simulink model "HANcoder_E407_TTA_Template_DS_V1"  (R2023a)
settings: Solver=FixedStepDiscrete  StartTime=0.0  StopTime=1  FixedStep=0.01  RelTol=1e-3
PreLoadFcn:
  | librarySetup
  | eval([bdroot,'_startup']) %Calling [modelName]_startup.m
values from neighbouring files (symbols this model uses):
  basic_cycle_duration_bc0 = TM_Reset_Board   + COMP_duration    (= 372)    [HANcoder_E407_TTA_Template_DS_V1_startup.m]    (also in HANcoder_E407_TTA_Template_DS_V2_startup.m; HANcoder_E407_TTA_Template_DS_V52_startup.m; HANcoder_E407_TTA_Template_DS_V5_startup.m; HANcoder_E407_TTA_Template_DS_V6_startup.m = 532)
  basic_cycle_duration_bc1 = basic_cycle_duration_bc0    (= 372)    [HANcoder_E407_TTA_Template_DS_V1_startup.m]    (also in HANcoder_E407_TTA_Template_DS_V2_startup.m; HANcoder_E407_TTA_Template_DS_V52_startup.m; HANcoder_E407_TTA_Template_DS_V5_startup.m; HANcoder_E407_TTA_Template_DS_V6_startup.m = 532)
  basic_cycle_duration_bc2 = basic_cycle_duration_bc0    (= 372)    [HANcoder_E407_TTA_Template_DS_V1_startup.m]    (also in HANcoder_E407_TTA_Template_DS_V2_startup.m; HANcoder_E407_TTA_Template_DS_V52_startup.m; HANcoder_E407_TTA_Template_DS_V5_startup.m; HANcoder_E407_TTA_Template_DS_V6_startup.m = 532)
  comm_delay_estimation1 = round(comm_delay_measured1*hardware_granularity/frequency_IRQ)    [HANcoder_E407_TTA_Template_DS_V1_startup.m]    (also in HANcoder_E407_TTA_Template_DS_V2_startup.m; HANcoder_E407_TTA_Template_DS_V52_startup.m; HANcoder_E407_TTA_Template_DS_V5_startup.m; HANcoder_E407_TTA_Template_DS_V6_startup.m)
  comm_delay_estimation2 = round(comm_delay_measured2*hardware_granularity/frequency_IRQ)    [HANcoder_E407_TTA_Template_DS_V1_startup.m]    (also in HANcoder_E407_TTA_Template_DS_V2_startup.m; HANcoder_E407_TTA_Template_DS_V52_startup.m; HANcoder_E407_TTA_Template_DS_V5_startup.m; HANcoder_E407_TTA_Template_DS_V6_startup.m)
  COMM_Period = 80    [HANcoder_E407_TTA_Template_DS_V1_startup.m]    (also in HANcoder_E407_TTA_Template_DS_V2_startup.m; HANcoder_E407_TTA_Template_DS_V52_startup.m; HANcoder_E407_TTA_Template_DS_V5_startup.m; HANcoder_E407_TTA_Template_DS_V6_startup.m = 120)
  COMM_Phase1 = Simulink.Parameter    [HANcoder_E407_TTA_Template_DS_V1_startup.m]    (also in HANcoder_E407_TTA_Template_DS_V2_startup.m; HANcoder_E407_TTA_Template_DS_V52_startup.m; HANcoder_E407_TTA_Template_DS_V5_startup.m; HANcoder_E407_TTA_Template_DS_V6_startup.m)
  COMM_Phase2 = Simulink.Parameter    [HANcoder_E407_TTA_Template_DS_V1_startup.m]    (also in HANcoder_E407_TTA_Template_DS_V2_startup.m; HANcoder_E407_TTA_Template_DS_V52_startup.m; HANcoder_E407_TTA_Template_DS_V5_startup.m; HANcoder_E407_TTA_Template_DS_V6_startup.m)
  COMM_Phase_init1 = Simulink.Parameter    [HANcoder_E407_TTA_Template_DS_V1_startup.m]    (also in HANcoder_E407_TTA_Template_DS_V2_startup.m; HANcoder_E407_TTA_Template_DS_V52_startup.m; HANcoder_E407_TTA_Template_DS_V5_startup.m; HANcoder_E407_TTA_Template_DS_V6_startup.m)
  COMM_Phase_init2 = Simulink.Parameter    [HANcoder_E407_TTA_Template_DS_V1_startup.m]    (also in HANcoder_E407_TTA_Template_DS_V2_startup.m; HANcoder_E407_TTA_Template_DS_V52_startup.m; HANcoder_E407_TTA_Template_DS_V5_startup.m; HANcoder_E407_TTA_Template_DS_V6_startup.m)
  COMP_duration = 4    [HANcoder_E407_TTA_Template_DS_V1_startup.m]    (also in HANcoder_E407_TTA_Template_DS_V2_startup.m; HANcoder_E407_TTA_Template_DS_V52_startup.m; HANcoder_E407_TTA_Template_DS_V5_startup.m; HANcoder_E407_TTA_Template_DS_V6_startup.m)
  frequency_IRQ = 100    [HANcoder_E407_TTA_Template_DS_V1_startup.m]    (also in HANcoder_E407_TTA_Template_DS_V2_startup.m; HANcoder_E407_TTA_Template_DS_V52_startup.m; HANcoder_E407_TTA_Template_DS_V5_startup.m; HANcoder_E407_TTA_Template_DS_V6_startup.m)
  idle_time_init = basic_cycle_duration_bc0 + basic_cycle_duration_bc1    (= 744)    [HANcoder_E407_TTA_Template_DS_V1_startup.m]    (also in HANcoder_E407_TTA_Template_DS_V2_startup.m; HANcoder_E407_TTA_Template_DS_V52_startup.m = 1116; HANcoder_E407_TTA_Template_DS_V5_startup.m = 1116; HANcoder_E407_TTA_Template_DS_V6_startup.m = 1596)
  LA_Clock_Gr = 1    [HANcoder_E407_TTA_Template_DS_V1_startup.m]    (also in HANcoder_E407_TTA_Template_DS_V2_startup.m; HANcoder_E407_TTA_Template_DS_V52_startup.m; HANcoder_E407_TTA_Template_DS_V5_startup.m; HANcoder_E407_TTA_Template_DS_V6_startup.m)
  LA_COMM_dly = 1    [HANcoder_E407_TTA_Template_DS_V1_startup.m]    (also in HANcoder_E407_TTA_Template_DS_V2_startup.m; HANcoder_E407_TTA_Template_DS_V52_startup.m; HANcoder_E407_TTA_Template_DS_V5_startup.m; HANcoder_E407_TTA_Template_DS_V6_startup.m)
  LA_COMM_Err = 1    [HANcoder_E407_TTA_Template_DS_V1_startup.m]    (also in HANcoder_E407_TTA_Template_DS_V2_startup.m; HANcoder_E407_TTA_Template_DS_V52_startup.m; HANcoder_E407_TTA_Template_DS_V5_startup.m; HANcoder_E407_TTA_Template_DS_V6_startup.m)
  LA_E_Desync = 1    [HANcoder_E407_TTA_Template_DS_V1_startup.m]    (also in HANcoder_E407_TTA_Template_DS_V2_startup.m; HANcoder_E407_TTA_Template_DS_V52_startup.m; HANcoder_E407_TTA_Template_DS_V5_startup.m; HANcoder_E407_TTA_Template_DS_V6_startup.m)
  LA_MEX_Flag = 1    [HANcoder_E407_TTA_Template_DS_V1_startup.m]    (also in HANcoder_E407_TTA_Template_DS_V2_startup.m; HANcoder_E407_TTA_Template_DS_V52_startup.m; HANcoder_E407_TTA_Template_DS_V5_startup.m; HANcoder_E407_TTA_Template_DS_V6_startup.m)
  LA_Task_Act = 1    [HANcoder_E407_TTA_Template_DS_V1_startup.m]    (also in HANcoder_E407_TTA_Template_DS_V2_startup.m; HANcoder_E407_TTA_Template_DS_V52_startup.m; HANcoder_E407_TTA_Template_DS_V5_startup.m; HANcoder_E407_TTA_Template_DS_V6_startup.m)
  Master_Role = 1    [HANcoder_E407_TTA_Template_DS_V1_startup.m]    (also in HANcoder_E407_TTA_Template_DS_V2_startup.m; HANcoder_E407_TTA_Template_DS_V52_startup.m; HANcoder_E407_TTA_Template_DS_V5_startup.m; HANcoder_E407_TTA_Template_DS_V6_startup.m)
  matrix_rows = 3    [HANcoder_E407_TTA_Template_DS_V1_startup.m]    (also in HANcoder_E407_TTA_Template_DS_V2_startup.m; HANcoder_E407_TTA_Template_DS_V52_startup.m; HANcoder_E407_TTA_Template_DS_V5_startup.m; HANcoder_E407_TTA_Template_DS_V6_startup.m)
  max_desync = 15    [HANcoder_E407_TTA_Template_DS_V1_startup.m]    (also in HANcoder_E407_TTA_Template_DS_V2_startup.m; HANcoder_E407_TTA_Template_DS_V52_startup.m; HANcoder_E407_TTA_Template_DS_V5_startup.m; HANcoder_E407_TTA_Template_DS_V6_startup.m)
  max_num_msgs_CAN1 = 2^Tx_bit_number-1    (= 7)    [HANcoder_E407_TTA_Template_DS_V1_startup.m]    (also in HANcoder_E407_TTA_Template_DS_V2_startup.m; HANcoder_E407_TTA_Template_DS_V52_startup.m; HANcoder_E407_TTA_Template_DS_V5_startup.m; HANcoder_E407_TTA_Template_DS_V6_startup.m)
  max_num_msgs_CAN2 = max_num_msgs_CAN1    (= 7)    [HANcoder_E407_TTA_Template_DS_V1_startup.m]    (also in HANcoder_E407_TTA_Template_DS_V2_startup.m; HANcoder_E407_TTA_Template_DS_V52_startup.m; HANcoder_E407_TTA_Template_DS_V5_startup.m; HANcoder_E407_TTA_Template_DS_V6_startup.m)
  min_desync = (-1)*max_desync    (= -15)    [HANcoder_E407_TTA_Template_DS_V1_startup.m]    (also in HANcoder_E407_TTA_Template_DS_V2_startup.m; HANcoder_E407_TTA_Template_DS_V52_startup.m; HANcoder_E407_TTA_Template_DS_V5_startup.m; HANcoder_E407_TTA_Template_DS_V6_startup.m)
  PotValue1_ID = 22    [HANcoder_E407_TTA_Template_DS_V1_startup.m]    (also in HANcoder_E407_TTA_Template_DS_V2_startup.m; HANcoder_E407_TTA_Template_DS_V52_startup.m; HANcoder_E407_TTA_Template_DS_V5_startup.m; HANcoder_E407_TTA_Template_DS_V6_startup.m)
  PotValue2_ID = 23    [HANcoder_E407_TTA_Template_DS_V1_startup.m]    (also in HANcoder_E407_TTA_Template_DS_V2_startup.m; HANcoder_E407_TTA_Template_DS_V52_startup.m; HANcoder_E407_TTA_Template_DS_V5_startup.m; HANcoder_E407_TTA_Template_DS_V6_startup.m)
  PotValue3_ID = 24    [HANcoder_E407_TTA_Template_DS_V1_startup.m]    (also in HANcoder_E407_TTA_Template_DS_V2_startup.m; HANcoder_E407_TTA_Template_DS_V52_startup.m; HANcoder_E407_TTA_Template_DS_V5_startup.m; HANcoder_E407_TTA_Template_DS_V6_startup.m)
  script_run = Simulink.Parameter    [HANcoder_E407_TTA_Template_DS_V1_startup.m]    (also in HANcoder_E407_TTA_Template_DS_V2_startup.m; HANcoder_E407_TTA_Template_DS_V52_startup.m; HANcoder_E407_TTA_Template_DS_V5_startup.m; HANcoder_E407_TTA_Template_DS_V6_startup.m)
  Slave_Role = 2    [HANcoder_E407_TTA_Template_DS_V1_startup.m]    (also in HANcoder_E407_TTA_Template_DS_V2_startup.m; HANcoder_E407_TTA_Template_DS_V52_startup.m; HANcoder_E407_TTA_Template_DS_V5_startup.m; HANcoder_E407_TTA_Template_DS_V6_startup.m)
  Sync_ID = 1    [HANcoder_E407_TTA_Template_DS_V1_startup.m]    (also in HANcoder_E407_TTA_Template_DS_V2_startup.m; HANcoder_E407_TTA_Template_DS_V52_startup.m; HANcoder_E407_TTA_Template_DS_V5_startup.m; HANcoder_E407_TTA_Template_DS_V6_startup.m)
  TM_Check_PotValue1 = TM_COMM_PotValue1 + COMM_duration    (= 174)    [HANcoder_E407_TTA_Template_DS_V1_startup.m]    (also in HANcoder_E407_TTA_Template_DS_V2_startup.m; HANcoder_E407_TTA_Template_DS_V52_startup.m; HANcoder_E407_TTA_Template_DS_V5_startup.m; HANcoder_E407_TTA_Template_DS_V6_startup.m = 254)
  TM_Check_PotValue2 = TM_COMM_PotValue2 + COMM_duration    (= 258)    [HANcoder_E407_TTA_Template_DS_V1_startup.m]    (also in HANcoder_E407_TTA_Template_DS_V2_startup.m; HANcoder_E407_TTA_Template_DS_V52_startup.m; HANcoder_E407_TTA_Template_DS_V5_startup.m; HANcoder_E407_TTA_Template_DS_V6_startup.m = 378)
  TM_Check_PotValue3 = TM_COMM_PotValue3 + COMM_duration    (= 342)    [HANcoder_E407_TTA_Template_DS_V1_startup.m]    (also in HANcoder_E407_TTA_Template_DS_V2_startup.m; HANcoder_E407_TTA_Template_DS_V52_startup.m; HANcoder_E407_TTA_Template_DS_V5_startup.m; HANcoder_E407_TTA_Template_DS_V6_startup.m = 502)
  TM_Check_Sync = TM_COMM_Sync   + COMM_duration    (= 80)    [HANcoder_E407_TTA_Template_DS_V1_startup.m]    (also in HANcoder_E407_TTA_Template_DS_V2_startup.m; HANcoder_E407_TTA_Template_DS_V52_startup.m; HANcoder_E407_TTA_Template_DS_V5_startup.m; HANcoder_E407_TTA_Template_DS_V6_startup.m = 120)
  TM_Check_TOuts = TM_Count_Vote3 + COMP_duration    (= 356)    [HANcoder_E407_TTA_Template_DS_V1_startup.m]    (also in HANcoder_E407_TTA_Template_DS_V2_startup.m; HANcoder_E407_TTA_Template_DS_V52_startup.m; HANcoder_E407_TTA_Template_DS_V5_startup.m; HANcoder_E407_TTA_Template_DS_V6_startup.m = 516)
  TM_Check_Trailer1Articulation = TM_COMM_Trailer1Articulation + COMM_duration    (= 170)    [HANcoder_E407_TTA_Template_DS_V1_startup.m]    (also in HANcoder_E407_TTA_Template_DS_V2_startup.m; HANcoder_E407_TTA_Template_DS_V52_startup.m; HANcoder_E407_TTA_Template_DS_V5_startup.m; HANcoder_E407_TTA_Template_DS_V6_startup.m = 250)
  TM_Check_Trailer2Articulation = TM_COMM_Trailer2Articulation + COMM_duration    (= 254)    [HANcoder_E407_TTA_Template_DS_V1_startup.m]    (also in HANcoder_E407_TTA_Template_DS_V2_startup.m; HANcoder_E407_TTA_Template_DS_V52_startup.m; HANcoder_E407_TTA_Template_DS_V5_startup.m; HANcoder_E407_TTA_Template_DS_V6_startup.m = 374)
  TM_Check_Vote1 = TM_COMM_Vote1  + COMM_duration    (= 172)    [HANcoder_E407_TTA_Template_DS_V1_startup.m]    (also in HANcoder_E407_TTA_Template_DS_V2_startup.m; HANcoder_E407_TTA_Template_DS_V52_startup.m; HANcoder_E407_TTA_Template_DS_V5_startup.m; HANcoder_E407_TTA_Template_DS_V6_startup.m = 252)
  TM_Check_Vote2 = TM_COMM_Vote2  + COMM_duration    (= 260)    [HANcoder_E407_TTA_Template_DS_V1_startup.m]    (also in HANcoder_E407_TTA_Template_DS_V2_startup.m; HANcoder_E407_TTA_Template_DS_V52_startup.m; HANcoder_E407_TTA_Template_DS_V5_startup.m; HANcoder_E407_TTA_Template_DS_V6_startup.m = 380)
  TM_Check_Vote3 = TM_COMM_Vote3  + COMM_duration    (= 348)    [HANcoder_E407_TTA_Template_DS_V1_startup.m]    (also in HANcoder_E407_TTA_Template_DS_V2_startup.m; HANcoder_E407_TTA_Template_DS_V52_startup.m; HANcoder_E407_TTA_Template_DS_V5_startup.m; HANcoder_E407_TTA_Template_DS_V6_startup.m = 508)
  TM_COMM_PotValue1 = TM_ReadPot + COMP_duration    (= 94)    [HANcoder_E407_TTA_Template_DS_V1_startup.m]    (also in HANcoder_E407_TTA_Template_DS_V2_startup.m; HANcoder_E407_TTA_Template_DS_V52_startup.m; HANcoder_E407_TTA_Template_DS_V5_startup.m; HANcoder_E407_TTA_Template_DS_V6_startup.m = 134)
  TM_COMM_PotValue2 = TM_Check_PotValue1 + COMP_duration    (= 178)    [HANcoder_E407_TTA_Template_DS_V1_startup.m]    (also in HANcoder_E407_TTA_Template_DS_V2_startup.m; HANcoder_E407_TTA_Template_DS_V52_startup.m; HANcoder_E407_TTA_Template_DS_V5_startup.m; HANcoder_E407_TTA_Template_DS_V6_startup.m = 258)
  TM_COMM_PotValue3 = TM_Check_PotValue2 + COMP_duration    (= 262)    [HANcoder_E407_TTA_Template_DS_V1_startup.m]    (also in HANcoder_E407_TTA_Template_DS_V2_startup.m; HANcoder_E407_TTA_Template_DS_V52_startup.m; HANcoder_E407_TTA_Template_DS_V5_startup.m; HANcoder_E407_TTA_Template_DS_V6_startup.m = 382)
  TM_COMM_Sync = basic_cycle_start    (= 0)    [HANcoder_E407_TTA_Template_DS_V1_startup.m]    (also in HANcoder_E407_TTA_Template_DS_V2_startup.m; HANcoder_E407_TTA_Template_DS_V52_startup.m; HANcoder_E407_TTA_Template_DS_V5_startup.m; HANcoder_E407_TTA_Template_DS_V6_startup.m)
  TM_COMM_Trailer1Articulation = TM_Update_LT_2 + COMP_duration    (= 90)    [HANcoder_E407_TTA_Template_DS_V1_startup.m]    (also in HANcoder_E407_TTA_Template_DS_V2_startup.m; HANcoder_E407_TTA_Template_DS_V52_startup.m; HANcoder_E407_TTA_Template_DS_V5_startup.m; HANcoder_E407_TTA_Template_DS_V6_startup.m = 130)
  TM_COMM_Trailer2Articulation = TM_Check_Trailer1Articulation + COMP_duration    (= 174)    [HANcoder_E407_TTA_Template_DS_V1_startup.m]    (also in HANcoder_E407_TTA_Template_DS_V2_startup.m; HANcoder_E407_TTA_Template_DS_V52_startup.m; HANcoder_E407_TTA_Template_DS_V5_startup.m; HANcoder_E407_TTA_Template_DS_V6_startup.m = 254)
  TM_COMM_Vote1 = TM_Vote_Dec    + COMP_duration    (= 92)    [HANcoder_E407_TTA_Template_DS_V1_startup.m]    (also in HANcoder_E407_TTA_Template_DS_V2_startup.m; HANcoder_E407_TTA_Template_DS_V52_startup.m; HANcoder_E407_TTA_Template_DS_V5_startup.m; HANcoder_E407_TTA_Template_DS_V6_startup.m = 132)
  TM_COMM_Vote2 = TM_Count_Vote1 + COMP_duration    (= 180)    [HANcoder_E407_TTA_Template_DS_V1_startup.m]    (also in HANcoder_E407_TTA_Template_DS_V2_startup.m; HANcoder_E407_TTA_Template_DS_V52_startup.m; HANcoder_E407_TTA_Template_DS_V5_startup.m; HANcoder_E407_TTA_Template_DS_V6_startup.m = 260)
  TM_COMM_Vote3 = TM_Count_Vote2 + COMP_duration    (= 268)    [HANcoder_E407_TTA_Template_DS_V1_startup.m]    (also in HANcoder_E407_TTA_Template_DS_V2_startup.m; HANcoder_E407_TTA_Template_DS_V52_startup.m; HANcoder_E407_TTA_Template_DS_V5_startup.m; HANcoder_E407_TTA_Template_DS_V6_startup.m = 388)
  TM_Count_Vote1 = TM_Check_Vote1 + COMP_duration    (= 176)    [HANcoder_E407_TTA_Template_DS_V1_startup.m]    (also in HANcoder_E407_TTA_Template_DS_V2_startup.m; HANcoder_E407_TTA_Template_DS_V52_startup.m; HANcoder_E407_TTA_Template_DS_V5_startup.m; HANcoder_E407_TTA_Template_DS_V6_startup.m = 256)
  TM_Count_Vote2 = TM_Check_Vote2 + COMP_duration    (= 264)    [HANcoder_E407_TTA_Template_DS_V1_startup.m]    (also in HANcoder_E407_TTA_Template_DS_V2_startup.m; HANcoder_E407_TTA_Template_DS_V52_startup.m; HANcoder_E407_TTA_Template_DS_V5_startup.m; HANcoder_E407_TTA_Template_DS_V6_startup.m = 384)
  TM_Count_Vote3 = TM_Check_Vote3 + COMP_duration    (= 352)    [HANcoder_E407_TTA_Template_DS_V1_startup.m]    (also in HANcoder_E407_TTA_Template_DS_V2_startup.m; HANcoder_E407_TTA_Template_DS_V52_startup.m; HANcoder_E407_TTA_Template_DS_V5_startup.m; HANcoder_E407_TTA_Template_DS_V6_startup.m = 512)
  TM_Data_bc0 = TM_COMM_Sync    (= 0)    [HANcoder_E407_TTA_Template_DS_V1_startup.m]    (also in HANcoder_E407_TTA_Template_DS_V2_startup.m; HANcoder_E407_TTA_Template_DS_V52_startup.m; HANcoder_E407_TTA_Template_DS_V5_startup.m; HANcoder_E407_TTA_Template_DS_V6_startup.m)
  TM_Data_bc1 = TM_Data_bc0(1:4)    [HANcoder_E407_TTA_Template_DS_V1_startup.m]    (also in HANcoder_E407_TTA_Template_DS_V2_startup.m; HANcoder_E407_TTA_Template_DS_V52_startup.m; HANcoder_E407_TTA_Template_DS_V5_startup.m; HANcoder_E407_TTA_Template_DS_V6_startup.m)
  TM_Data_bc2 = TM_Data_bc0(1:4)    [HANcoder_E407_TTA_Template_DS_V1_startup.m]    (also in HANcoder_E407_TTA_Template_DS_V2_startup.m; HANcoder_E407_TTA_Template_DS_V52_startup.m; HANcoder_E407_TTA_Template_DS_V5_startup.m; HANcoder_E407_TTA_Template_DS_V6_startup.m)
  TM_New_Master = TM_Check_TOuts + COMP_duration    (= 360)    [HANcoder_E407_TTA_Template_DS_V1_startup.m]    (also in HANcoder_E407_TTA_Template_DS_V2_startup.m; HANcoder_E407_TTA_Template_DS_V52_startup.m; HANcoder_E407_TTA_Template_DS_V5_startup.m; HANcoder_E407_TTA_Template_DS_V6_startup.m = 520)
  TM_PotVote = TM_COMM_PotValue3 + COMP_duration    (= 266)    [HANcoder_E407_TTA_Template_DS_V1_startup.m]    (also in HANcoder_E407_TTA_Template_DS_V2_startup.m; HANcoder_E407_TTA_Template_DS_V52_startup.m; HANcoder_E407_TTA_Template_DS_V5_startup.m; HANcoder_E407_TTA_Template_DS_V6_startup.m = 386)
  TM_ReadPot = TM_Update_LT_2 + COMP_duration    (= 90)    [HANcoder_E407_TTA_Template_DS_V1_startup.m]    (also in HANcoder_E407_TTA_Template_DS_V2_startup.m; HANcoder_E407_TTA_Template_DS_V52_startup.m; HANcoder_E407_TTA_Template_DS_V5_startup.m; HANcoder_E407_TTA_Template_DS_V6_startup.m = 130)
  TM_Reset_Board = TM_Reset_Var   + COMP_duration    (= 368)    [HANcoder_E407_TTA_Template_DS_V1_startup.m]    (also in HANcoder_E407_TTA_Template_DS_V2_startup.m; HANcoder_E407_TTA_Template_DS_V52_startup.m; HANcoder_E407_TTA_Template_DS_V5_startup.m; HANcoder_E407_TTA_Template_DS_V6_startup.m = 528)
  TM_Reset_Var = TM_New_Master  + COMP_duration    (= 364)    [HANcoder_E407_TTA_Template_DS_V1_startup.m]    (also in HANcoder_E407_TTA_Template_DS_V2_startup.m; HANcoder_E407_TTA_Template_DS_V52_startup.m; HANcoder_E407_TTA_Template_DS_V5_startup.m; HANcoder_E407_TTA_Template_DS_V6_startup.m = 524)
  TM_Reset_Var_bc1 = TM_Data_bc1(end) + COMP_duration    [HANcoder_E407_TTA_Template_DS_V1_startup.m]    (also in HANcoder_E407_TTA_Template_DS_V2_startup.m; HANcoder_E407_TTA_Template_DS_V52_startup.m; HANcoder_E407_TTA_Template_DS_V5_startup.m; HANcoder_E407_TTA_Template_DS_V6_startup.m)
  TM_Reset_Var_bc1_2 = TM_Reset_Var_bc1 +2    [HANcoder_E407_TTA_Template_DS_V1_startup.m]    (also in HANcoder_E407_TTA_Template_DS_V2_startup.m; HANcoder_E407_TTA_Template_DS_V52_startup.m; HANcoder_E407_TTA_Template_DS_V5_startup.m; HANcoder_E407_TTA_Template_DS_V6_startup.m)
  TM_Type_bc0 = COMM    (= 0)    [HANcoder_E407_TTA_Template_DS_V1_startup.m]    (also in HANcoder_E407_TTA_Template_DS_V2_startup.m; HANcoder_E407_TTA_Template_DS_V52_startup.m; HANcoder_E407_TTA_Template_DS_V5_startup.m; HANcoder_E407_TTA_Template_DS_V6_startup.m)
  TM_Type_bc1 = TM_Type_bc0(1:4)    [HANcoder_E407_TTA_Template_DS_V1_startup.m]    (also in HANcoder_E407_TTA_Template_DS_V2_startup.m; HANcoder_E407_TTA_Template_DS_V52_startup.m; HANcoder_E407_TTA_Template_DS_V5_startup.m; HANcoder_E407_TTA_Template_DS_V6_startup.m)
  TM_Type_bc2 = TM_Type_bc0(1:4)    [HANcoder_E407_TTA_Template_DS_V1_startup.m]    (also in HANcoder_E407_TTA_Template_DS_V2_startup.m; HANcoder_E407_TTA_Template_DS_V52_startup.m; HANcoder_E407_TTA_Template_DS_V5_startup.m; HANcoder_E407_TTA_Template_DS_V6_startup.m)
  TM_Update_LT = TM_Check_Sync  + COMP_duration    (= 84)    [HANcoder_E407_TTA_Template_DS_V1_startup.m]    (also in HANcoder_E407_TTA_Template_DS_V2_startup.m; HANcoder_E407_TTA_Template_DS_V52_startup.m; HANcoder_E407_TTA_Template_DS_V5_startup.m; HANcoder_E407_TTA_Template_DS_V6_startup.m = 124)
  TM_Update_LT_2 = TM_Update_LT   + 2    (= 86)    [HANcoder_E407_TTA_Template_DS_V1_startup.m]    (also in HANcoder_E407_TTA_Template_DS_V2_startup.m; HANcoder_E407_TTA_Template_DS_V52_startup.m; HANcoder_E407_TTA_Template_DS_V5_startup.m; HANcoder_E407_TTA_Template_DS_V6_startup.m = 126)
  TM_Vote_Dec = TM_Update_LT   + COMP_duration    (= 88)    [HANcoder_E407_TTA_Template_DS_V1_startup.m]    (also in HANcoder_E407_TTA_Template_DS_V2_startup.m; HANcoder_E407_TTA_Template_DS_V52_startup.m; HANcoder_E407_TTA_Template_DS_V5_startup.m; HANcoder_E407_TTA_Template_DS_V6_startup.m = 128)
  Tractor_Board1 = 11    [HANcoder_E407_TTA_Template_DS_V1_startup.m]    (also in HANcoder_E407_TTA_Template_DS_V2_startup.m = 1; HANcoder_E407_TTA_Template_DS_V52_startup.m = 1; HANcoder_E407_TTA_Template_DS_V5_startup.m = 1; HANcoder_E407_TTA_Template_DS_V6_startup.m = 1)
  Trailer1_Articulation_ID = 31    [HANcoder_E407_TTA_Template_DS_V1_startup.m]    (also in HANcoder_E407_TTA_Template_DS_V2_startup.m; HANcoder_E407_TTA_Template_DS_V52_startup.m; HANcoder_E407_TTA_Template_DS_V5_startup.m; HANcoder_E407_TTA_Template_DS_V6_startup.m)
  Trailer1_Board1 = 2    [HANcoder_E407_TTA_Template_DS_V1_startup.m]    (also in HANcoder_E407_TTA_Template_DS_V2_startup.m = 4; HANcoder_E407_TTA_Template_DS_V52_startup.m = 4; HANcoder_E407_TTA_Template_DS_V5_startup.m = 4; HANcoder_E407_TTA_Template_DS_V6_startup.m = 4)
  Trailer1_Board2 = 3    [HANcoder_E407_TTA_Template_DS_V1_startup.m]    (also in HANcoder_E407_TTA_Template_DS_V2_startup.m = 5; HANcoder_E407_TTA_Template_DS_V52_startup.m = 5; HANcoder_E407_TTA_Template_DS_V5_startup.m = 5; HANcoder_E407_TTA_Template_DS_V6_startup.m = 5)
  Trailer1_Board3 = 4    [HANcoder_E407_TTA_Template_DS_V1_startup.m]    (also in HANcoder_E407_TTA_Template_DS_V2_startup.m = 6; HANcoder_E407_TTA_Template_DS_V52_startup.m = 6; HANcoder_E407_TTA_Template_DS_V5_startup.m = 6; HANcoder_E407_TTA_Template_DS_V6_startup.m = 6)
  Trailer2_Articulation_ID = 32    [HANcoder_E407_TTA_Template_DS_V1_startup.m]    (also in HANcoder_E407_TTA_Template_DS_V2_startup.m; HANcoder_E407_TTA_Template_DS_V52_startup.m; HANcoder_E407_TTA_Template_DS_V5_startup.m; HANcoder_E407_TTA_Template_DS_V6_startup.m)
  Trailer2_Board1 = 5    [HANcoder_E407_TTA_Template_DS_V1_startup.m]    (also in HANcoder_E407_TTA_Template_DS_V2_startup.m = 7; HANcoder_E407_TTA_Template_DS_V52_startup.m = 7; HANcoder_E407_TTA_Template_DS_V5_startup.m = 7; HANcoder_E407_TTA_Template_DS_V6_startup.m = 7)
  Trailer2_Board2 = 6    [HANcoder_E407_TTA_Template_DS_V1_startup.m]    (also in HANcoder_E407_TTA_Template_DS_V2_startup.m = 8; HANcoder_E407_TTA_Template_DS_V52_startup.m = 8; HANcoder_E407_TTA_Template_DS_V5_startup.m = 8; HANcoder_E407_TTA_Template_DS_V6_startup.m = 8)
  Trailer2_Board3 = 7    [HANcoder_E407_TTA_Template_DS_V1_startup.m]    (also in HANcoder_E407_TTA_Template_DS_V2_startup.m = 9; HANcoder_E407_TTA_Template_DS_V52_startup.m = 9; HANcoder_E407_TTA_Template_DS_V5_startup.m = 9; HANcoder_E407_TTA_Template_DS_V6_startup.m = 9)
  Vote1_ID = 11    [HANcoder_E407_TTA_Template_DS_V1_startup.m]    (also in HANcoder_E407_TTA_Template_DS_V2_startup.m; HANcoder_E407_TTA_Template_DS_V52_startup.m; HANcoder_E407_TTA_Template_DS_V5_startup.m; HANcoder_E407_TTA_Template_DS_V6_startup.m)
  Vote2_ID = 12    [HANcoder_E407_TTA_Template_DS_V1_startup.m]    (also in HANcoder_E407_TTA_Template_DS_V2_startup.m; HANcoder_E407_TTA_Template_DS_V52_startup.m; HANcoder_E407_TTA_Template_DS_V5_startup.m; HANcoder_E407_TTA_Template_DS_V6_startup.m)
  Vote3_ID = 13    [HANcoder_E407_TTA_Template_DS_V1_startup.m]    (also in HANcoder_E407_TTA_Template_DS_V2_startup.m; HANcoder_E407_TTA_Template_DS_V52_startup.m; HANcoder_E407_TTA_Template_DS_V5_startup.m; HANcoder_E407_TTA_Template_DS_V6_startup.m)
undefined symbols (not defined in the file or in its folder): A0, A1, A2, A3, A4, A5, CON2, CON4, D10, D12, D13, D8, D9
libraries: hdlsllib x164, HANcoder_STM32_Target x28, simulink x12, simulink_extras x1, dspstat3 x1
(part 5 of 34)

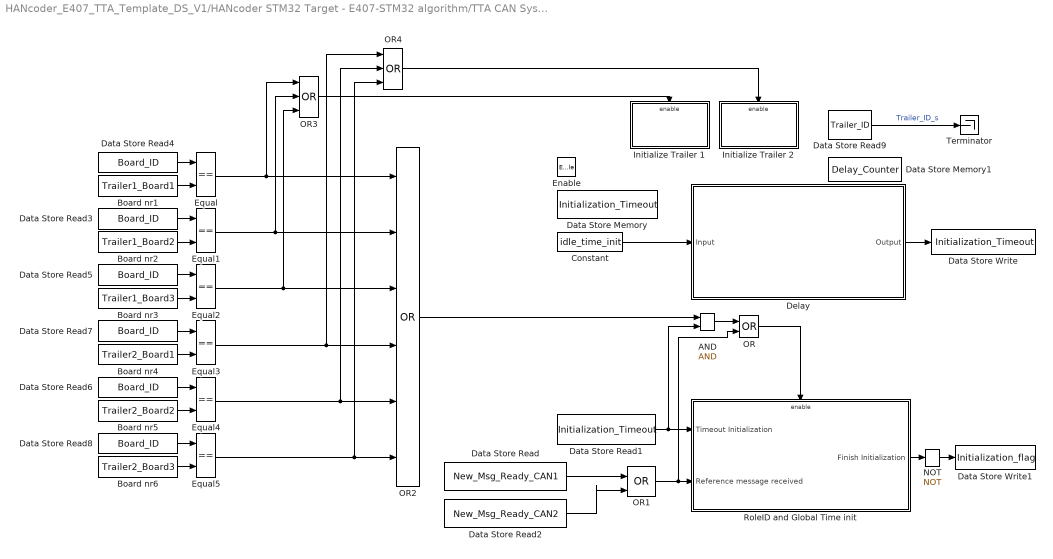
== system HANcoder_E407_TTA_Template_DS_V1/HANcoder STM32 Target - E407-STM32 algorithm/TTA CAN System/TTA System/Initialization ==
  Enable : EnablePort  PropagateVarSize=During execution
  AND : Logic  IconShape=distinctive  AllPortsSameDT=off  OutDataTypeStr=boolean
  Board nr1 : Constant  Value=Trailer1_Board1
  Board nr2 : Constant  Value=Trailer1_Board2
  Board nr3 : Constant  Value=Trailer1_Board3
  Board nr4 : Constant  Value=Trailer2_Board1
  Board nr5 : Constant  Value=Trailer2_Board2
  Board nr6 : Constant  Value=Trailer2_Board3
  Constant : Constant  Value=idle_time_init
  Data Store Memory : DataStoreMemory  DataStoreName=Initialization_Timeout  ReadBeforeWriteMsg=warning  WriteAfterWriteMsg=warning  WriteAfterReadMsg=warning  ShowAdditionalParam=off  OutDataTypeStr=boolean
  Data Store Memory1 : DataStoreMemory  DataStoreName=Delay_Counter  ReadBeforeWriteMsg=warning  WriteAfterWriteMsg=warning  WriteAfterReadMsg=warning  ShowAdditionalParam=off  OutDataTypeStr=double
  Data Store Read : DataStoreRead  DataStoreName=New_Msg_Ready_CAN1  IndexOptions=Index vector (dialog)  Indices=1  OutputSizes=1
  Data Store Read1 : DataStoreRead  DataStoreName=Initialization_Timeout  IndexOptions=Index vector (dialog)  Indices=1  OutputSizes=1
  Data Store Read2 : DataStoreRead  DataStoreName=New_Msg_Ready_CAN2  IndexOptions=Index vector (dialog)  Indices=1  OutputSizes=1
  Data Store Read{3..8} (6 alike) : DataStoreRead  DataStoreName=Board_ID  IndexOptions=Index vector (dialog)  Indices=1  OutputSizes=1
  Data Store Read9 : DataStoreRead  DataStoreName=Trailer_ID  IndexOptions=Index vector (dialog)  Indices=1  OutputSizes=1
  Data Store Write : DataStoreWrite  DataStoreName=Initialization_Timeout  IndexOptions=Index vector (dialog)  Indices=1  OutputSizes=1
  Data Store Write1 : DataStoreWrite  DataStoreName=Initialization_flag  IndexOptions=Index vector (dialog)  Indices=1  OutputSizes=1
  Delay : Subsystem
  Equal{,1..5} (6 alike) : RelationalOperator  Operator===  OutDataTypeStr=boolean  RndMeth=Simplest  InputSameDT=off
  Initialize Trailer 1 : Subsystem  TreatAsAtomicUnit=on
  Initialize Trailer 2 : Subsystem  TreatAsAtomicUnit=on
  NOT : Logic  Operator=NOT  IconShape=distinctive  AllPortsSameDT=off  OutDataTypeStr=boolean
  OR : Logic  Operator=OR  IconShape=distinctive  AllPortsSameDT=off  OutDataTypeStr=boolean
  OR1 : Logic  Operator=OR  IconShape=distinctive  AllPortsSameDT=off  OutDataTypeStr=boolean
  OR2 : Logic  Operator=OR  Inputs=6  IconShape=distinctive  AllPortsSameDT=off  OutDataTypeStr=boolean
  OR3 : Logic  Operator=OR  Inputs=3  IconShape=distinctive  AllPortsSameDT=off  OutDataTypeStr=boolean
  OR4 : Logic  Operator=OR  Inputs=3  IconShape=distinctive  AllPortsSameDT=off  OutDataTypeStr=boolean
  RoleID and Global Time init : Subsystem  TreatAsAtomicUnit=on
  Terminator : Terminator
  wires:
  Delay/1(Output) -> Data Store Write/1
  Constant/1 -> Delay/1(Input)
  NOT/1 -> Data Store Write1/1
  RoleID and Global Time init/1(Finish Initialization) -> NOT/1
  OR/1 -> RoleID and Global Time init/Enable
  Data Store Read1/1 -> AND/2, RoleID and Global Time init/1(Timeout Initialization)
  OR1/1 -> OR/2, RoleID and Global Time init/2(Reference message received)
  Data Store Read4/1 -> Equal/1
  Board nr1/1 -> Equal/2
  OR2/1 -> AND/1
  AND/1 -> OR/1
  Data Store Read/1 -> OR1/1
  Data Store Read2/1 -> OR1/2
  Equal/1 -> OR3/1, OR2/1
  Equal1/1 -> OR3/2, OR2/2
  Equal2/1 -> OR3/3, OR2/3
  Board nr2/1 -> Equal1/2
  Data Store Read3/1 -> Equal1/1
  Board nr3/1 -> Equal2/2
  Data Store Read5/1 -> Equal2/1
  OR3/1 -> Initialize Trailer 1/Enable
  Board nr5/1 -> Equal4/2
  Data Store Read6/1 -> Equal4/1
  Data Store Read8/1 -> Equal5/1
  Board nr6/1 -> Equal5/2
  Board nr4/1 -> Equal3/2
  Data Store Read7/1 -> Equal3/1
  Equal3/1 -> OR4/1, OR2/4
  Equal4/1 -> OR4/2, OR2/5
  Equal5/1 -> OR4/3, OR2/6
  OR4/1 -> Initialize Trailer 2/Enable
  Data Store Read9/1 -> Terminator/1  "Trailer_ID_s"

== system HANcoder_E407_TTA_Template_DS_V1/HANcoder STM32 Target - E407-STM32 algorithm/TTA CAN System/TTA System/LT_Update Desync_Positive ==
  note: Local Time Update with Positive Desync
      | This subsystem is only activated if we have to update
      | the local time with a positive desync. This is activated
      | at the end of the current Computational Task, so the
      | Local Time is updated until the tick before the next
      | Computational Task in the basic cycle. This way we
      | avoid missing tasks, as would happened when updating
      | the Local Time too quickly into the future.
  note: WARNING
      | TM_Type is currently defined as
      | COMM type 0
      | COMP type 1
  note: Constants bc0
  note: constants are defined in the _startup file
  note: Constants bc1
  note: Constants bc2
  Local Time : Inport
  Bacic_Cycle : Inport  Port=2
  Enable : EnablePort  PropagateVarSize=During execution
  Bus Selector : BusSelector  OutputSignals=signal1,signal2
  Bus Creator : BusCreator  Inputs=2
  Bus Creator1 : BusCreator  Inputs=2
  Bus Creator2 : BusCreator  Inputs=2
  Constant : Constant  Value=TM_Data_bc0
  Constant1 : Constant  Value=TM_Type_bc0
  Constant10 : Constant  Value=TM_Data_bc2
  Constant11 : Constant  Value=TM_Type_bc2
  Constant2 : Constant  Value=COMM_Phase1
  Constant3 : Constant  Value=COMM_Phase2
  Constant4 : Constant  Value=TM_Data_bc1
  Constant5 : Constant  Value=TM_Type_bc1
  Constant6 : Constant  Value=COMM_Phase_init1
  Constant7 : Constant  Value=COMM_Phase_init2
  Constant8 : Constant  Value=0
  Constant9 : Constant
  Equal : RelationalOperator  Operator===  OutDataTypeStr=boolean  RndMeth=Simplest  InputSameDT=off
  Equal1 : RelationalOperator  Operator===  OutDataTypeStr=boolean  RndMeth=Simplest  InputSameDT=off
  Local Time Update with Positive Desync : Subsystem  TreatAsAtomicUnit=on
  MATLAB Function : MATLAB Function  TreatAsAtomicUnit=on
  Switch : Switch  Criteria=u2 > Threshold  AllowDiffInputSizes=on  SaturateOnIntegerOverflow=off  InputSameDT=off
  Switch1 : Switch  Criteria=u2 > Threshold  AllowDiffInputSizes=on  SaturateOnIntegerOverflow=off  InputSameDT=off
  wires:
  MATLAB Function/1(result_time) -> Local Time Update with Positive Desync/1(Ticks until next COMP)
  Local Time/1 -> MATLAB Function/1(local_time)
  Constant8/1 -> Equal/2
  Equal/1 -> Switch/2
  Constant/1 -> Bus Creator/1
  Constant1/1 -> Bus Creator/2
  Bus Creator/1 -> Switch/1
  Constant4/1 -> Bus Creator1/1
  Constant5/1 -> Bus Creator1/2
  Switch/1 -> Bus Selector/1
  Bus Selector/1 -> MATLAB Function/2(TM_data)  "<signal1>"
  Bus Selector/2 -> MATLAB Function/3(TM_type)  "<signal2>"
  Constant3/1 -> MATLAB Function/7(phase2)
  Constant2/1 -> MATLAB Function/5(phase1)
  Constant6/1 -> MATLAB Function/4(phase_init1)
  Constant7/1 -> MATLAB Function/6(phase_init2)
  Bus Creator1/1 -> Switch1/1
  Switch1/1 -> Switch/3
  Bacic_Cycle/1 -> Equal1/1, Equal/1
  Constant9/1 -> Equal1/2
  Equal1/1 -> Switch1/2
  Constant10/1 -> Bus Creator2/1
  Constant11/1 -> Bus Creator2/2
  Bus Creator2/1 -> Switch1/3

== system HANcoder_E407_TTA_Template_DS_V1/HANcoder STM32 Target - E407-STM32 algorithm/TTA CAN System/TTA System/Logic Analyzer - COMM delay CAN1 - Rx ==
  note: Change pin state
  note: Reset
  Enable : EnablePort
  Constant : Constant  OutDataTypeStr=boolean
  Constant1 : Constant  Value=0  OutDataTypeStr=boolean
  Constant2 : Constant  Value=0
  Data Store Read : DataStoreRead  DataStoreName=D12_Pin_State  IndexOptions=Index vector (dialog)  Indices=1  OutputSizes=1
  Data Store Read1 : DataStoreRead  Priority=2  DataStoreName=D12_Pin_State  IndexOptions=Index vector (dialog)  Indices=1  OutputSizes=1
  Data Store Write1 : DataStoreWrite  Priority=1  DataStoreName=D12_Pin_State  IndexOptions=Index vector (dialog)  Indices=1  OutputSizes=1
  Data Store Write2 : DataStoreWrite  Priority=3  DataStoreName=Toggle_Pin_D12  IndexOptions=Index vector (dialog)  Indices=1  OutputSizes=1
  Digital Output : HANcoder_STM32_Target/STM32-E407/Digital Outputs/Digital Output  Tag=HANcoder_TARGET_STM32_E407  pinID=CON4 - D12  config=Open drain  tsamp=-1
      settings: SourceProductName=HANcoder STM32 Target
  Switch : Switch  Criteria=u2 > Threshold  SaturateOnIntegerOverflow=off  InputSameDT=off
  wires:
  Data Store Read/1 -> Switch/2
  Data Store Read1/1 -> Digital Output/1
  Constant1/1 -> Switch/1
  Constant/1 -> Switch/3
  Switch/1 -> Data Store Write1/1
  Constant2/1 -> Data Store Write2/1

== system HANcoder_E407_TTA_Template_DS_V1/HANcoder STM32 Target - E407-STM32 algorithm/TTA CAN System/TTA System/Logic Analyzer - COMM delay CAN1 - Tx ==
  note: Reset
  note: Change pin state
  Enable : EnablePort
  Constant : Constant  OutDataTypeStr=boolean
  Constant1 : Constant  Value=0  OutDataTypeStr=boolean
  Constant2 : Constant  Value=0
  Data Store Read : DataStoreRead  DataStoreName=D13_Pin_State  IndexOptions=Index vector (dialog)  Indices=1  OutputSizes=1
  Data Store Read1 : DataStoreRead  Priority=2  DataStoreName=D13_Pin_State  IndexOptions=Index vector (dialog)  Indices=1  OutputSizes=1
  Data Store Write1 : DataStoreWrite  Priority=1  DataStoreName=D13_Pin_State  IndexOptions=Index vector (dialog)  Indices=1  OutputSizes=1
  Data Store Write2 : DataStoreWrite  Priority=3  DataStoreName=Toggle_Pin_D13  IndexOptions=Index vector (dialog)  Indices=1  OutputSizes=1
  Digital Output : HANcoder_STM32_Target/STM32-E407/Digital Outputs/Digital Output  Tag=HANcoder_TARGET_STM32_E407  pinID=CON4 - D13  config=Open drain  tsamp=-1
      settings: SourceProductName=HANcoder STM32 Target
  Switch : Switch  Criteria=u2 > Threshold  SaturateOnIntegerOverflow=off  InputSameDT=off
  wires:
  Switch/1 -> Data Store Write1/1
  Constant/1 -> Switch/3
  Constant1/1 -> Switch/1
  Data Store Read1/1 -> Digital Output/1
  Data Store Read/1 -> Switch/2
  Constant2/1 -> Data Store Write2/1

== system HANcoder_E407_TTA_Template_DS_V1/HANcoder STM32 Target - E407-STM32 algorithm/TTA CAN System/TTA System/Logic Analyzer - COMM delay CAN2 - Rx ==
  note: Change pin state
  note: Reset
  Enable : EnablePort
  Constant : Constant  OutDataTypeStr=boolean
  Constant1 : Constant  Value=0  OutDataTypeStr=boolean
  Constant2 : Constant  Value=0
  Data Store Read : DataStoreRead  DataStoreName=D8_Pin_State  IndexOptions=Index vector (dialog)  Indices=1  OutputSizes=1
  Data Store Read1 : DataStoreRead  Priority=2  DataStoreName=D8_Pin_State  IndexOptions=Index vector (dialog)  Indices=1  OutputSizes=1
  Data Store Write1 : DataStoreWrite  Priority=1  DataStoreName=D8_Pin_State  IndexOptions=Index vector (dialog)  Indices=1  OutputSizes=1
  Data Store Write2 : DataStoreWrite  Priority=3  DataStoreName=Toggle_Pin_D8  IndexOptions=Index vector (dialog)  Indices=1  OutputSizes=1
  Digital Output : HANcoder_STM32_Target/STM32-E407/Digital Outputs/Digital Output  Tag=HANcoder_TARGET_STM32_E407  pinID=CON4 - D8  config=Open drain  tsamp=-1
      settings: SourceProductName=HANcoder STM32 Target
  Switch : Switch  Criteria=u2 > Threshold  SaturateOnIntegerOverflow=off  InputSameDT=off
  wires:
  Data Store Read/1 -> Switch/2
  Data Store Read1/1 -> Digital Output/1
  Constant1/1 -> Switch/1
  Constant/1 -> Switch/3
  Switch/1 -> Data Store Write1/1
  Constant2/1 -> Data Store Write2/1

== system HANcoder_E407_TTA_Template_DS_V1/HANcoder STM32 Target - E407-STM32 algorithm/TTA CAN System/TTA System/Logic Analyzer - COMM delay CAN2 - Tx ==
  note: Change pin state
  note: Reset
  Enable : EnablePort
  Constant : Constant  OutDataTypeStr=boolean
  Constant1 : Constant  Value=0  OutDataTypeStr=boolean
  Constant2 : Constant  Value=0
  Data Store Read : DataStoreRead  DataStoreName=D9_Pin_State  IndexOptions=Index vector (dialog)  Indices=1  OutputSizes=1
  Data Store Read1 : DataStoreRead  Priority=2  DataStoreName=D9_Pin_State  IndexOptions=Index vector (dialog)  Indices=1  OutputSizes=1
  Data Store Write1 : DataStoreWrite  Priority=1  DataStoreName=D9_Pin_State  IndexOptions=Index vector (dialog)  Indices=1  OutputSizes=1
  Data Store Write2 : DataStoreWrite  Priority=3  DataStoreName=Toggle_Pin_D9  IndexOptions=Index vector (dialog)  Indices=1  OutputSizes=1
  Digital Output : HANcoder_STM32_Target/STM32-E407/Digital Outputs/Digital Output  Tag=HANcoder_TARGET_STM32_E407  pinID=CON4 - D9  config=Open drain  tsamp=-1
      settings: SourceProductName=HANcoder STM32 Target
  Switch : Switch  Criteria=u2 > Threshold  SaturateOnIntegerOverflow=off  InputSameDT=off
  wires:
  Switch/1 -> Data Store Write1/1
  Constant/1 -> Switch/3
  Constant1/1 -> Switch/1
  Data Store Read1/1 -> Digital Output/1
  Data Store Read/1 -> Switch/2
  Constant2/1 -> Data Store Write2/1

== system HANcoder_E407_TTA_Template_DS_V1/HANcoder STM32 Target - E407-STM32 algorithm/TTA CAN System/TTA System/Matrix Cycle Manager ==
  note: Controller boards condition
  note: Output Send_Message
      | Send: 1
      | Do not send: 0
  note: Output Receive_Message
      | Receive: 1
      | Do not receive: 0
  note: Output Receive_Message
      | Receive: 1
      | Do not receive: 0
  note: Output Send_Message
      | Send: 1
      | Do not send: 0
  Enable : EnablePort  PropagateVarSize=During execution
  Constant : Constant  Value=Trailer1_Board1
  Constant1 : Constant  Value=Trailer1_Board2
  Constant2 : Constant  Value=Trailer1_Board3
  Constant3 : Constant  Value=Trailer2_Board1
  Constant4 : Constant  Value=Trailer2_Board2
  Constant5 : Constant  Value=Trailer2_Board3
  Controller Matrix Cycle : Subsystem
  Data Store Read : DataStoreRead  DataStoreName=Board_ID  IndexOptions=Index vector (dialog)  Indices=1  OutputSizes=1
  Data Store Read10 : DataStoreRead  DataStoreName=basic_cycle_count  IndexOptions=Index vector (dialog)  Indices=1  OutputSizes=1
  Equal{,1..5} (6 alike) : RelationalOperator  Operator===  OutDataTypeStr=boolean  RndMeth=Simplest  InputSameDT=off
  OR : Logic  Operator=OR  Inputs=6  IconShape=distinctive  AllPortsSameDT=off  OutDataTypeStr=boolean
  Send_Message_CAN1 : Outport  OutputWhenDisabled=reset  InitialOutput=0  VectorParamsAs1DForOutWhenUnconnected=off
  Send_Message_CAN2 : Outport  Port=2  OutputWhenDisabled=reset  InitialOutput=0  VectorParamsAs1DForOutWhenUnconnected=off
  Receive_Message_CAN1 : Outport  Port=3  OutputWhenDisabled=reset  InitialOutput=0  VectorParamsAs1DForOutWhenUnconnected=off
  Receive_Message_CAN2 : Outport  Port=4  OutputWhenDisabled=reset  InitialOutput=0  VectorParamsAs1DForOutWhenUnconnected=off
  wires:
  Constant/1 -> Equal/2
  Constant1/1 -> Equal1/2
  Constant2/1 -> Equal2/2
  OR/1 -> Controller Matrix Cycle/Enable
  Controller Matrix Cycle/4(Receive_CAN2) -> Receive_Message_CAN2/1
  Controller Matrix Cycle/3(Receive_CAN1) -> Receive_Message_CAN1/1
  Controller Matrix Cycle/2(Send_CAN2) -> Send_Message_CAN2/1
  Controller Matrix Cycle/1(Send_CAN1) -> Send_Message_CAN1/1
  Data Store Read10/1 -> Controller Matrix Cycle/1(basic_cycle)
  Constant5/1 -> Equal5/2
  Constant4/1 -> Equal4/2
  Data Store Read/1 -> Equal3/1, Equal5/1, Equal4/1, Equal2/1, Equal1/1, Equal/1
  Constant3/1 -> Equal3/2
  Equal/1 -> OR/1
  Equal2/1 -> OR/3
  Equal3/1 -> OR/4
  Equal4/1 -> OR/5
  Equal5/1 -> OR/6
  Equal1/1 -> OR/2

== system HANcoder_E407_TTA_Template_DS_V1/HANcoder STM32 Target - E407-STM32 algorithm/TTA CAN System/CAN1 Recieve/RxID_CAN/PotValue1_ID_CAN ==
  Enable : EnablePort
  CAN receive1 : Subsystem  Tag=HANcoder_TARGET_STM32_E407  AncestorBlock=HANcoder_STM32_Target/STM32-E407/CAN/CAN/CAN receive  mask(CAN receive){canBus=CAN 1, outputNumber=8, dataType=uint8, byteOrder=off, tsamp=-1}
      mask prompts: canBus "CAN channel"; outputNumber "Output ports"; dataType "Output datatype"; byteOrder "Byte order: Checked = MSB first, unchecked = LSB first."; tsamp "Sample time"
      mask help:
      | Function
      | ==========
      | Receive the newest message from the specified CAN channel.
      |
      | Parameters
      | ==========
      | CAN channel:             The CAN channel to send the message on.
      | Output ports:             The amount of output ports
      | Output datatype:       The datatype of the output ports
      | Byte order:                 Select MSB or LSB first
      | Sample time:              -1 or divisible by base sample time [seconds]
      |
      | Input
      | ==========
      | Port 1:                       CAN ID(uint32) in hexadecimal ie: hex2dec('0a')
      |
      | Output
      | ==========
      | Port 1:                       Checks for new message(int8)
      | Port 2..9                     Message data
      mask init:
      | sfcn_can_receive_mcb(canBus, outputNumber, dataType, byteOrder)
      settings: LibrarySourceBlock=HANcoder_STM32_Target/STM32-E407/CAN/CAN/CAN receive  MoveFcn=drawLogos
      mask Help: web('sfcn_can_receive.html');
      mask TypeOptions canBus: CAN 1 | CAN 2
      mask TypeOptions dataType: int8 | uint8 | int16 | uint16 | int32 | uint32 | boolean
      mask Display:
      | fprintf('Receive on\nCAN %x', canBus);
      | port_label('output', 1, 'new');
      | port_label('input', 1, 'ID');patch([135 141 141],[8 14 2],[1 0 0]);patch([143 143 149],[14 2 8],[0 0 0.35]);
  Constant3 : Constant  Value=PotValue1_ID  OutDataTypeStr=uint32
  CAN_new : Outport  OutputWhenDisabled=reset  InitialOutput=0  VectorParamsAs1DForOutWhenUnconnected=off
  Out2 : Outport  Port=2  OutputWhenDisabled=reset  InitialOutput=0  VectorParamsAs1DForOutWhenUnconnected=off
  Out3 : Outport  Port=3  OutputWhenDisabled=reset  InitialOutput=0  VectorParamsAs1DForOutWhenUnconnected=off
  Out4 : Outport  Port=4  OutputWhenDisabled=reset  InitialOutput=0  VectorParamsAs1DForOutWhenUnconnected=off
  Out5 : Outport  Port=5  OutputWhenDisabled=reset  InitialOutput=0  VectorParamsAs1DForOutWhenUnconnected=off
  Out6 : Outport  Port=6  OutputWhenDisabled=reset  InitialOutput=0  VectorParamsAs1DForOutWhenUnconnected=off
  Out7 : Outport  Port=7  OutputWhenDisabled=reset  InitialOutput=0  VectorParamsAs1DForOutWhenUnconnected=off
  Out8 : Outport  Port=8  OutputWhenDisabled=reset  InitialOutput=0  VectorParamsAs1DForOutWhenUnconnected=off
  Out9 : Outport  Port=9  OutputWhenDisabled=reset  InitialOutput=0  VectorParamsAs1DForOutWhenUnconnected=off
  wires:
  Constant3/1 -> CAN receive1/1(In1)
  CAN receive1/9(Out9) -> Out9/1
  CAN receive1/5(Out5) -> Out5/1
  CAN receive1/4(Out4) -> Out4/1
  CAN receive1/7(Out7) -> Out7/1
  CAN receive1/6(Out6) -> Out6/1
  CAN receive1/2(Out2) -> Out2/1
  CAN receive1/3(Out3) -> Out3/1
  CAN receive1/8(Out8) -> Out8/1
  CAN receive1/1(Out1) -> CAN_new/1

== system HANcoder_E407_TTA_Template_DS_V1/HANcoder STM32 Target - E407-STM32 algorithm/TTA CAN System/CAN1 Recieve/RxID_CAN/PotValue2_ID_CAN ==
  Enable : EnablePort
  CAN receive1 : Subsystem  Tag=HANcoder_TARGET_STM32_E407  AncestorBlock=HANcoder_STM32_Target/STM32-E407/CAN/CAN/CAN receive  mask(CAN receive){canBus=CAN 1, outputNumber=8, dataType=uint8, byteOrder=off, tsamp=-1}
      mask prompts: canBus "CAN channel"; outputNumber "Output ports"; dataType "Output datatype"; byteOrder "Byte order: Checked = MSB first, unchecked = LSB first."; tsamp "Sample time"
      mask help:
      | Function
      | ==========
      | Receive the newest message from the specified CAN channel.
      |
      | Parameters
      | ==========
      | CAN channel:             The CAN channel to send the message on.
      | Output ports:             The amount of output ports
      | Output datatype:       The datatype of the output ports
      | Byte order:                 Select MSB or LSB first
      | Sample time:              -1 or divisible by base sample time [seconds]
      |
      | Input
      | ==========
      | Port 1:                       CAN ID(uint32) in hexadecimal ie: hex2dec('0a')
      |
      | Output
      | ==========
      | Port 1:                       Checks for new message(int8)
      | Port 2..9                     Message data
      mask init:
      | sfcn_can_receive_mcb(canBus, outputNumber, dataType, byteOrder)
      settings: LibrarySourceBlock=HANcoder_STM32_Target/STM32-E407/CAN/CAN/CAN receive  MoveFcn=drawLogos
      mask Help: web('sfcn_can_receive.html');
      mask TypeOptions canBus: CAN 1 | CAN 2
      mask TypeOptions dataType: int8 | uint8 | int16 | uint16 | int32 | uint32 | boolean
      mask Display:
      | fprintf('Receive on\nCAN %x', canBus);
      | port_label('output', 1, 'new');
      | port_label('input', 1, 'ID');patch([135 141 141],[8 14 2],[1 0 0]);patch([143 143 149],[14 2 8],[0 0 0.35]);
  Constant3 : Constant  Value=PotValue1_ID*2  OutDataTypeStr=uint32
  CAN_new : Outport  OutputWhenDisabled=reset  InitialOutput=0  VectorParamsAs1DForOutWhenUnconnected=off
  Out2 : Outport  Port=2  OutputWhenDisabled=reset  InitialOutput=0  VectorParamsAs1DForOutWhenUnconnected=off
  Out3 : Outport  Port=3  OutputWhenDisabled=reset  InitialOutput=0  VectorParamsAs1DForOutWhenUnconnected=off
  Out4 : Outport  Port=4  OutputWhenDisabled=reset  InitialOutput=0  VectorParamsAs1DForOutWhenUnconnected=off
  Out5 : Outport  Port=5  OutputWhenDisabled=reset  InitialOutput=0  VectorParamsAs1DForOutWhenUnconnected=off
  Out6 : Outport  Port=6  OutputWhenDisabled=reset  InitialOutput=0  VectorParamsAs1DForOutWhenUnconnected=off
  Out7 : Outport  Port=7  OutputWhenDisabled=reset  InitialOutput=0  VectorParamsAs1DForOutWhenUnconnected=off
  Out8 : Outport  Port=8  OutputWhenDisabled=reset  InitialOutput=0  VectorParamsAs1DForOutWhenUnconnected=off
  Out9 : Outport  Port=9  OutputWhenDisabled=reset  InitialOutput=0  VectorParamsAs1DForOutWhenUnconnected=off
  wires:
  Constant3/1 -> CAN receive1/1(In1)
  CAN receive1/9(Out9) -> Out9/1
  CAN receive1/5(Out5) -> Out5/1
  CAN receive1/4(Out4) -> Out4/1
  CAN receive1/7(Out7) -> Out7/1
  CAN receive1/6(Out6) -> Out6/1
  CAN receive1/2(Out2) -> Out2/1
  CAN receive1/3(Out3) -> Out3/1
  CAN receive1/8(Out8) -> Out8/1
  CAN receive1/1(Out1) -> CAN_new/1

== system HANcoder_E407_TTA_Template_DS_V1/HANcoder STM32 Target - E407-STM32 algorithm/TTA CAN System/CAN1 Recieve/RxID_CAN/PotValue2_ID_CAN1 ==
  Enable : EnablePort
  CAN receive1 : Subsystem  Tag=HANcoder_TARGET_STM32_E407  AncestorBlock=HANcoder_STM32_Target/STM32-E407/CAN/CAN/CAN receive  mask(CAN receive){canBus=CAN 1, outputNumber=8, dataType=uint8, byteOrder=off, tsamp=-1}
      mask prompts: canBus "CAN channel"; outputNumber "Output ports"; dataType "Output datatype"; byteOrder "Byte order: Checked = MSB first, unchecked = LSB first."; tsamp "Sample time"
      mask help:
      | Function
      | ==========
      | Receive the newest message from the specified CAN channel.
      |
      | Parameters
      | ==========
      | CAN channel:             The CAN channel to send the message on.
      | Output ports:             The amount of output ports
      | Output datatype:       The datatype of the output ports
      | Byte order:                 Select MSB or LSB first
      | Sample time:              -1 or divisible by base sample time [seconds]
      |
      | Input
      | ==========
      | Port 1:                       CAN ID(uint32) in hexadecimal ie: hex2dec('0a')
      |
      | Output
      | ==========
      | Port 1:                       Checks for new message(int8)
      | Port 2..9                     Message data
      mask init:
      | sfcn_can_receive_mcb(canBus, outputNumber, dataType, byteOrder)
      settings: LibrarySourceBlock=HANcoder_STM32_Target/STM32-E407/CAN/CAN/CAN receive  MoveFcn=drawLogos
      mask Help: web('sfcn_can_receive.html');
      mask TypeOptions canBus: CAN 1 | CAN 2
      mask TypeOptions dataType: int8 | uint8 | int16 | uint16 | int32 | uint32 | boolean
      mask Display:
      | fprintf('Receive on\nCAN %x', canBus);
      | port_label('output', 1, 'new');
      | port_label('input', 1, 'ID');patch([135 141 141],[8 14 2],[1 0 0]);patch([143 143 149],[14 2 8],[0 0 0.35]);
  Constant3 : Constant  Value=PotValue2_ID  OutDataTypeStr=uint32
  CAN_new : Outport  OutputWhenDisabled=reset  InitialOutput=0  VectorParamsAs1DForOutWhenUnconnected=off
  Out2 : Outport  Port=2  OutputWhenDisabled=reset  InitialOutput=0  VectorParamsAs1DForOutWhenUnconnected=off
  Out3 : Outport  Port=3  OutputWhenDisabled=reset  InitialOutput=0  VectorParamsAs1DForOutWhenUnconnected=off
  Out4 : Outport  Port=4  OutputWhenDisabled=reset  InitialOutput=0  VectorParamsAs1DForOutWhenUnconnected=off
  Out5 : Outport  Port=5  OutputWhenDisabled=reset  InitialOutput=0  VectorParamsAs1DForOutWhenUnconnected=off
  Out6 : Outport  Port=6  OutputWhenDisabled=reset  InitialOutput=0  VectorParamsAs1DForOutWhenUnconnected=off
  Out7 : Outport  Port=7  OutputWhenDisabled=reset  InitialOutput=0  VectorParamsAs1DForOutWhenUnconnected=off
  Out8 : Outport  Port=8  OutputWhenDisabled=reset  InitialOutput=0  VectorParamsAs1DForOutWhenUnconnected=off
  Out9 : Outport  Port=9  OutputWhenDisabled=reset  InitialOutput=0  VectorParamsAs1DForOutWhenUnconnected=off
  wires:
  CAN receive1/9(Out9) -> Out9/1
  CAN receive1/5(Out5) -> Out5/1
  CAN receive1/4(Out4) -> Out4/1
  CAN receive1/7(Out7) -> Out7/1
  CAN receive1/6(Out6) -> Out6/1
  CAN receive1/2(Out2) -> Out2/1
  CAN receive1/3(Out3) -> Out3/1
  CAN receive1/8(Out8) -> Out8/1
  CAN receive1/1(Out1) -> CAN_new/1
  Constant3/1 -> CAN receive1/1(In1)
